simulink model "steering_control2"  (R2020b)
settings: Solver=VariableStepAuto  StartTime=0.0  StopTime=10.0  RelTol=1e-3
model workspace (MAT data in the model file):
  ROBOT_L = 0.14
  c = 0
  m = 1
  update_time = 0.02
undefined symbols (not defined in the file or in its folder): DiscIntNeverNeededParam, sample_time, sigbuilder_block
libraries: simulink x4, dspstat3 x1
settings Model: Creator=ped02  LastModifiedBy=ped02

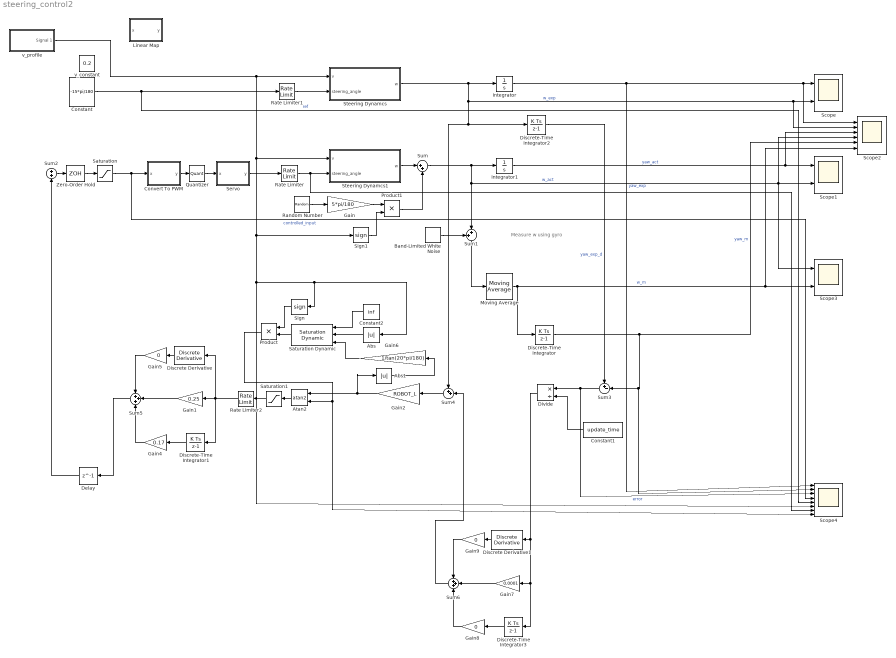
== system steering_control2 ==
  note: Measure w using gyro
  Abs : Abs
  Abs1 : Abs
  Atan2 : Trigonometry  Operator=atan2
  Band-Limited White Noise : simulink/Sources/Band-Limited White Noise  Cov=[0.015]  Ts=0.01  seed=[23341]
  Constant : Constant  Value=-15*pi/180
  Constant1 : Constant  Value=update_time
  Constant2 : Constant  Value=inf
  Convert To PWM : Subsystem  mask{m=-97.7486, c=148}
      mask prompts: m "Gain"; c "Offset"
  Delay : Delay  DelayLength=1  SampleTime=update_time
  Discrete Derivative : simulink/Discrete/Discrete Derivative  gainval=1.0  ICPrevScaledInput=0.0  OutMin=[]  OutMax=[]  OutDataType=fixdt(1, 16)  OutScaling=2^-10  DoSatur=off
  Discrete Derivative1 : simulink/Discrete/Discrete Derivative  gainval=1.0  ICPrevScaledInput=0.0  OutMin=[]  OutMax=[]  OutDataType=fixdt(1, 16)  OutScaling=2^-10  DoSatur=off
  Discrete-Time Integrator{,1..3} (4 alike) : DiscreteIntegrator  SampleTime=sample_time  ICPrevOutput=DiscIntNeverNeededParam  ICPrevScaledInput=DiscIntNeverNeededParam
  Divide : Product  Inputs=*/
  Gain : Gain  Gain=5*pi/180
  Gain1 : Gain  Gain=0.25
  Gain2 : Gain  Gain=ROBOT_L
  Gain4 : Gain  Gain=0.17
  Gain5 : Gain  Gain=0
  Gain6 : Gain  Gain=1/tan(20*pi/180)
  Gain7 : Gain  Gain=0.0001
  Gain8 : Gain  Gain=0
  Gain9 : Gain  Gain=0
  Integrator : Integrator
  Integrator1 : Integrator
  Linear Map : Subsystem  mask{m=1, c=0}
      mask prompts: m "Gain"; c "Offset"
  Moving Average : dspstat3/Moving Average  Method=Sliding window  ForgettingFactorPort=off  SpecifyWindowLength=on  WindowLength=5  ForgettingFactor=0.9  SimulateUsing=Code generation
  Product : Product
  Product1 : Product
  Quantizer : Quantizer  QuantizationInterval=1
  Random Number : RandomNumber  SampleTime=0.5
  Rate Limiter : RateLimiter  RisingSlewLimit=pi/4  FallingSlewLimit=-pi/4  SampleTimeMode=inherited
  Rate Limiter1 : RateLimiter  RisingSlewLimit=pi/4  FallingSlewLimit=-pi/4  SampleTimeMode=inherited
  Rate Limiter2 : RateLimiter  RisingSlewLimit=pi/4  FallingSlewLimit=-pi/4  SampleTimeMode=inherited
  Saturation : Saturate  UpperLimit=20*pi/180  LowerLimit=-20*pi/180
  Saturation Dynamic : simulink/Discontinuities/Saturation Dynamic  OutMin=[]  OutMax=[]  OutDataTypeStr=Inherit: Same as second input  OutDataType=fixdt(1, 16)  OutScaling=2^-10  DoSatur=off
  Saturation1 : Saturate  UpperLimit=20*pi/180  LowerLimit=-20*pi/180
  Scope : Scope  NumInputPorts=2
  Scope1 : Scope  NumInputPorts=2
  Scope2 : Scope  NumInputPorts=6
  Scope3 : Scope  NumInputPorts=2
  Scope4 : Scope  NumInputPorts=8
  Servo : Subsystem  mask{m=-1/75, c=146.3/75}
      mask prompts: m "Gain"; c "Offset"
  Sign : Signum
  Sign1 : Signum
  Steering Dynamcs : Subsystem
  Steering Dynamcs1 : Subsystem
  Sum : Sum  Inputs=|++
  Sum1 : Sum  Inputs=++|
  Sum2 : Sum  Inputs=+|+
  Sum3 : Sum  Inputs=+-|
  Sum4 : Sum  Inputs=++|
  Sum5 : Sum  Inputs=+++
  Sum6 : Sum  Inputs=+++
  Zero-Order Hold : ZeroOrderHold  SampleTime=update_time
  v_constant : Constant  Value=0.2
  v_profile : Subsystem  Tag=STV Subsys  LoadFcn=sigbuilder_block('load');  StartFcn=sigbuilder_block('start');  StopFcn=sigbuilder_block('stop');  ClipboardFcn=sigbuilder_block('clipboard');  mask(Sigbuilder block){tuvar=[0:10]}
      mask help: Simulink:masks:SigbuilderBlock_MD
      mask init:
      | if ~strcmp(get_param(bdroot(gcbh),'SimulationStatus'),'stopped') tuvar = sigbuilder_block('maskInit'); end
      settings: CopyFcn=sigbuilder_block('copy');  DeleteFcn=sigbuilder_block('delete');  ModelCloseFcn=sigbuilder_block('modelClose');  PreSaveFcn=sigbuilder_block('preSave');  PauseFcn=sigbuilder_block('pause');  ContinueFcn=sigbuilder_block('continue');  NameChangeFcn=sigbuilder_block('namechange');  OpenFcn=sigbuilder_block('open',[437.6 199.2 550.4 400 ]);  CloseFcn=sigbuilder_block('close');
      mask Display: plot(0, 0, 100, 100,[2, 2, 32, 32, 2], [68, 8, 8, 68, 68],[32, 2], [38, 38], [32, 19, 2],[53, 60, 44], [32, 17, 17, 2],[16, 16, 31, 31]);txt = getActiveGroup(gcbh);text(2, 100, txt,'verticalAlignment', 'top');
  wires:
  Steering Dynamcs/1(w) -> Discrete-Time Integrator2/1, Sum4/1, Scope2/2, Scope/2, Integrator/1  "w_exp"
  Integrator/1 -> Scope4/1, Scope2/1, Scope/1  "yaw_exp"
  Integrator1/1 -> Scope2/3, Scope1/1  "yaw_act"
  Gain/1 -> Product1/1
  Random Number/1 -> Gain/1
  Band-Limited White Noise/1 -> Sum1/1
  Sum1/1 -> Moving Average/1
  Servo/1(y) -> Rate Limiter/1
  Sum/1 -> Sum1/2, Scope3/1, Scope2/4, Scope1/2, Integrator1/1  "w_act"
  Steering Dynamcs1/1(w) -> Sum/1
  Moving Average/1 -> Discrete-Time Integrator/1, Scope3/2, Scope2/6  "w_m"
  Discrete-Time Integrator/1 -> Scope4/2, Sum3/2, Scope2/5  "yaw_m"
  Sum2/1 -> Zero-Order Hold/1
  Discrete-Time Integrator2/1 -> Sum3/1  "yaw_exp_d"
  Constant1/1 -> Divide/2
  Convert To PWM/1(y) -> Quantizer/1
  Sum3/1 -> Scope4/3, Divide/1  "error"
  Atan2/1 -> Saturation1/1
  Sum4/1 -> Gain2/1
  Gain2/1 -> Abs1/1, Atan2/1
  Zero-Order Hold/1 -> Saturation/1
  Quantizer/1 -> Servo/1(x)
  Saturation/1 -> Scope4/4, Convert To PWM/1(x)  "controlled_input"
  Rate Limiter/1 -> Scope4/7, Steering Dynamcs1/2(steering_angle)
  Rate Limiter1/1 -> Steering Dynamcs/2(steering_angle)
  Constant/1 -> Scope4/5, Rate Limiter1/1  "ref"
  v_profile/1(Signal 1) -> Sign1/1, Scope4/6, Sign/1, Abs/1, Steering Dynamcs1/1(v), Steering Dynamcs/1(v)
  Gain1/1 -> Sum5/2
  Discrete-Time Integrator1/1 -> Gain4/1
  Gain4/1 -> Sum5/3
  Delay/1 -> Sum2/2
  Sum5/1 -> Delay/1
  Saturation1/1 -> Rate Limiter2/1
  Discrete Derivative/1 -> Gain5/1
  Gain5/1 -> Sum5/1
  Rate Limiter2/1 -> Discrete-Time Integrator1/1, Discrete Derivative/1, Gain1/1
  Constant2/1 -> Saturation Dynamic/1
  Abs/1 -> Saturation Dynamic/2
  Gain6/1 -> Saturation Dynamic/3
  Saturation Dynamic/1 -> Product/2
  Sign/1 -> Product/1
  Product/1 -> Scope4/8, Atan2/2
  Abs1/1 -> Gain6/1
  Product1/1 -> Sum/2
  Sign1/1 -> Product1/2
  Gain9/1 -> Sum6/1
  Discrete Derivative1/1 -> Gain9/1
  Gain8/1 -> Sum6/3
  Discrete-Time Integrator3/1 -> Gain8/1
  Gain7/1 -> Sum6/2
  Sum6/1 -> Sum4/2
  Divide/1 -> Discrete Derivative1/1, Discrete-Time Integrator3/1, Gain7/1

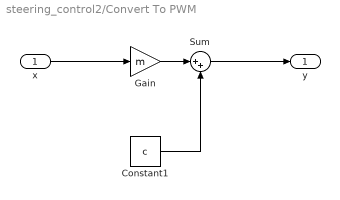
== system steering_control2/Convert To PWM ==
  x : Inport
  Constant1 : Constant  Value=c
  Gain : Gain  Gain=m
  Sum : Sum  Inputs=|++
  y : Outport
  wires:
  Gain/1 -> Sum/1
  Constant1/1 -> Sum/2
  x/1 -> Gain/1
  Sum/1 -> y/1

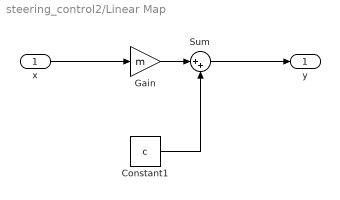
== system steering_control2/Linear Map ==
  x : Inport
  Constant1 : Constant  Value=c
  Gain : Gain  Gain=m
  Sum : Sum  Inputs=|++
  y : Outport
  wires:
  Sum/1 -> y/1
  x/1 -> Gain/1
  Constant1/1 -> Sum/2
  Gain/1 -> Sum/1

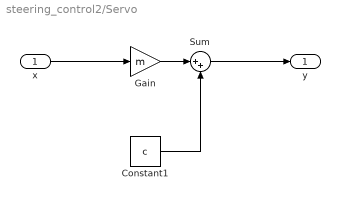
== system steering_control2/Servo ==
  x : Inport
  Constant1 : Constant  Value=c
  Gain : Gain  Gain=m
  Sum : Sum  Inputs=|++
  y : Outport
  wires:
  Sum/1 -> y/1
  x/1 -> Gain/1
  Constant1/1 -> Sum/2
  Gain/1 -> Sum/1

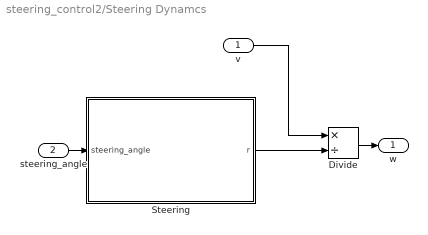
== system steering_control2/Steering Dynamcs ==
  v : Inport
  steering_angle : Inport  Port=2
  Divide : Product  Inputs=*/
  Steering : Subsystem
  w : Outport
  wires:
  steering_angle/1 -> Steering/1(steering_angle)
  Steering/1(r) -> Divide/2
  Divide/1 -> w/1
  v/1 -> Divide/1

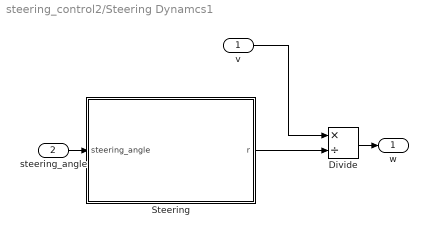
== system steering_control2/Steering Dynamcs1 ==
  v : Inport
  steering_angle : Inport  Port=2
  Divide : Product  Inputs=*/
  Steering : Subsystem
  w : Outport
  wires:
  v/1 -> Divide/1
  Divide/1 -> w/1
  Steering/1(r) -> Divide/2
  steering_angle/1 -> Steering/1(steering_angle)

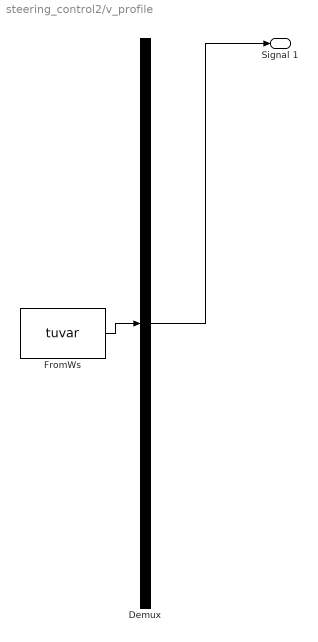
== system steering_control2/v_profile ==
  Demux : Demux  Tag=STV Demux  Outputs=1
      settings: DisplayOption=none
  FromWs : FromWorkspace  Tag=STV FromWs  VariableName=tuvar
      SigBuilderData=|
      | common.afterFinalStr = 'Extrapolate'
      | common.sampleTime = 0
      | dataSet.timeRange = [0 10]
      | dataSet.name = 'Group 1'
      | sbobj.Groups.Name = 'Group 1'
      | sbobj.Groups.Signals.Name = 'Signal 1'
      | sbobj.Groups.Signals.XData = [0 0.5 1.5 4 5 10]
      | sbobj.Groups.Signals.YData = [0 0 0.2 0.2 0 0]
  Signal 1 : Outport  Tag=STV Outport
  wires:
  Demux/1 -> Signal 1/1
  FromWs/1 -> Demux/1

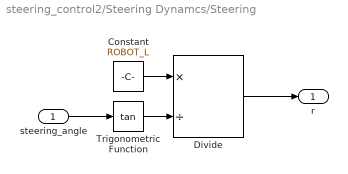
== system steering_control2/Steering Dynamcs/Steering ==
  steering_angle : Inport
  Constant : Constant  Value=ROBOT_L
  Divide : Product  Inputs=*/
  Trigonometric Function : Trigonometry  Operator=tan
  r : Outport
  wires:
  Trigonometric Function/1 -> Divide/2
  steering_angle/1 -> Trigonometric Function/1
  Constant/1 -> Divide/1
  Divide/1 -> r/1

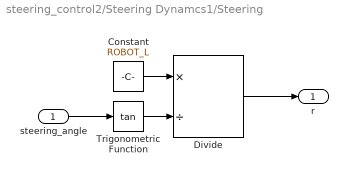
== system steering_control2/Steering Dynamcs1/Steering ==
  steering_angle : Inport
  Constant : Constant  Value=ROBOT_L
  Divide : Product  Inputs=*/
  Trigonometric Function : Trigonometry  Operator=tan
  r : Outport
  wires:
  Divide/1 -> r/1
  Constant/1 -> Divide/1
  steering_angle/1 -> Trigonometric Function/1
  Trigonometric Function/1 -> Divide/2
